simulink model "sampleModel1536"  (R2023a)
settings: Solver=VariableStepAuto  StartTime=0.0  StopTime=10.0  RelTol=1e-3
libraries: hdlsllib x6, simulink x2
settings Model: Creator=user1  LastModifiedBy=user1

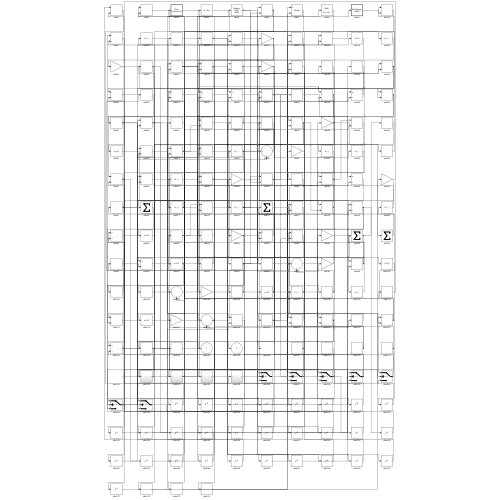
[thumbnail: Simulink's stored preview of the top-level diagram]
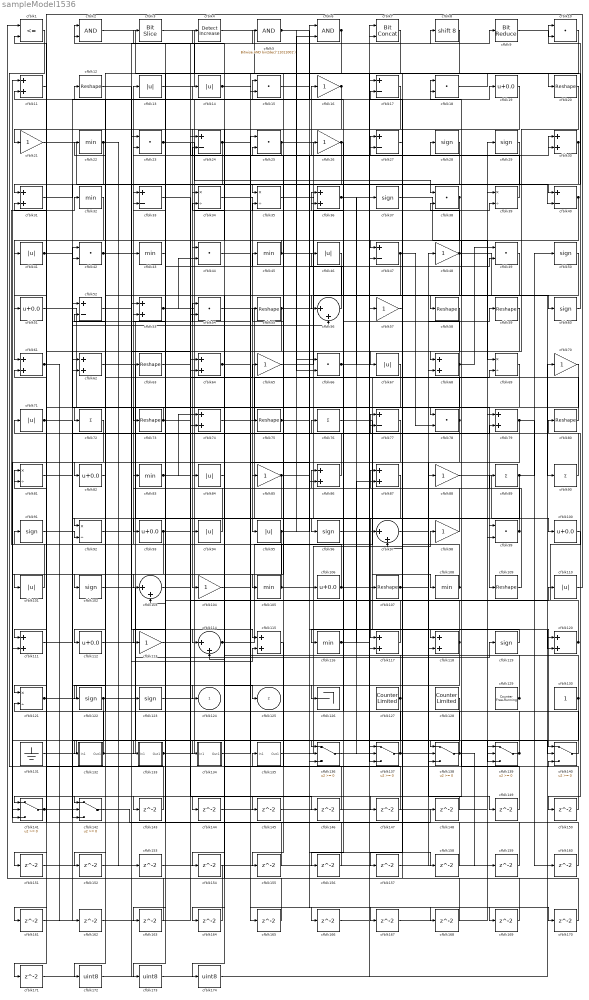
== system sampleModel1536 ==
  cfblk1 : RelationalOperator  Operator=<=  OutDataTypeStr=boolean  InputSameDT=off
  cfblk{10,15,18,23,25,38,42,44,49,54,66,78,99} (13 alike) : DotProduct  OutDataTypeStr=Inherit: Inherit via internal rule
  cfblk{19,51,82,93,100,106,112} (7 alike) : Bias  Bias=0.0  SaturateOnIntegerOverflow=off
  cfblk{13..14,41,46,67,71,84,94..95,101,110} (11 alike) : Abs  SaturateOnIntegerOverflow=off
  cfblk{28..29,37,50,60,91,96,102,119,122..123} (11 alike) : Signum
  cfblk{56,97,103,114} (4 alike) : Sum  Inputs=|++
  cfblk{16,21,26,48,57,65,70,85,88,98,104,113} (12 alike) : Gain
  cfblk{22,32,43,45,83,105,108,116} (8 alike) : MinMax
  cfblk{12,20,55,58..59,63,73,75,80,107,109} (11 alike) : Reshape
  cfblk{11,30..31,36,53,61..62,64,68,74,79,86..87,111,115,117..118,120} (18 alike) : Sum
  cfblk{34..35,39,69,81,92,121} (7 alike) : Product  Inputs=*/  RndMeth=Zero  SaturateOnIntegerOverflow=on
  cfblk126 : Terminator
  cfblk127 : hdlsllib/Sources/Counter Limited  uplimit=7  tsamp=-1
  cfblk128 : hdlsllib/Sources/Counter Limited  uplimit=7  tsamp=-1
  cfblk129 : hdlsllib/Sources/Counter Free-Running  NumBits=16  tsamp=-1
  cfblk130 : Constant  SampleTime=-1
  cfblk131 : Ground
  cfblk132 : Subsystem
      settings: LibrarySourceBlock=|
      | hdlsllib/Ports &
      | Subsystems/Subsystem
  cfblk133 : Subsystem
      settings: LibrarySourceBlock=|
      | hdlsllib/Ports &
      | Subsystems/Subsystem
  cfblk134 : Subsystem
      settings: LibrarySourceBlock=|
      | hdlsllib/Ports &
      | Subsystems/Subsystem
  cfblk135 : Subsystem
      settings: LibrarySourceBlock=|
      | hdlsllib/Ports &
      | Subsystems/Subsystem
  cfblk{136..142} (7 alike) : Switch  SaturateOnIntegerOverflow=off  InputSameDT=off
  cfblk{143..171} (29 alike) : Delay  SampleTime=1
  cfblk{17,24,27,33,40,47,52,77} (8 alike) : Sum  Inputs=+-
  cfblk172 : DataTypeConversion  OutDataTypeStr=uint8  SaturateOnIntegerOverflow=off  RndMeth=Floor
  cfblk173 : DataTypeConversion  OutDataTypeStr=uint8  SaturateOnIntegerOverflow=off  RndMeth=Floor
  cfblk174 : DataTypeConversion  OutDataTypeStr=uint8  SaturateOnIntegerOverflow=off  RndMeth=Floor
  cfblk2 : Logic  AllPortsSameDT=off  OutDataTypeStr=boolean
  cfblk3 : hdlsllib/Logic and Bit Operations/Bit Slice  lidx=7  ridx=0
  cfblk4 : simulink/Logic and Bit Operations/Detect Increase  vinit=0.0  OutDataTypeStr=boolean
      settings: LibrarySourceBlock=|
      | hdlsllib/Logic and Bit
      | Operations/Detect
      | Increase
  cfblk5 : simulink/Logic and Bit Operations/Bitwise Operator  logicop=AND  UseBitMask=on  BitMask=bin2dec('11011001')  BitMaskRealWorld=Stored Integer
      settings: LibrarySourceBlock=|
      | hdlsllib/Logic and Bit
      | Operations/Bitwise
      | Operator
  cfblk6 : Logic  AllPortsSameDT=off  OutDataTypeStr=boolean
  cfblk7 : hdlsllib/Logic and Bit Operations/Bit Concat  numInputs=2
  cfblk{72,76,89..90} (4 alike) : Sum  Inputs=+
  cfblk8 : ArithShift  BitShiftNumber=8
  cfblk9 : hdlsllib/Logic and Bit Operations/Bit Reduce  mode=AND
  cfblk124 : Outport  VectorParamsAs1DForOutWhenUnconnected=off
  cfblk125 : Outport  Port=2  VectorParamsAs1DForOutWhenUnconnected=off
  wires:
  cfblk86/1 -> cfblk71/1
  cfblk34/1 -> cfblk95/1
  cfblk122/1 -> cfblk138/1, cfblk115/2, cfblk171/1
  cfblk101/1 -> cfblk32/1
  cfblk21/1 -> cfblk35/1
  cfblk66/1 -> cfblk37/1, cfblk69/2
  cfblk73/1 -> cfblk72/1, cfblk138/2
  cfblk32/1 -> cfblk111/1
  cfblk39/1 -> cfblk16/1
  cfblk76/1 -> cfblk118/1
  cfblk105/1 -> cfblk13/1, cfblk120/2
  cfblk55/1 -> cfblk78/1, cfblk151/1, cfblk158/1
  cfblk54/1 -> cfblk117/1
  cfblk112/1 -> cfblk119/1
  cfblk20/1 -> cfblk68/1
  cfblk1/1 -> cfblk135/1(In1)
  cfblk2/1 -> cfblk40/1
  cfblk49/1 -> cfblk92/1
  cfblk23/1 -> cfblk38/1, cfblk6/1, cfblk30/2
  cfblk51/1 -> cfblk109/1
  cfblk130/1 -> cfblk142/1, cfblk2/2
  cfblk82/1 -> cfblk12/1
  cfblk96/1 -> cfblk108/1
  cfblk127/1 -> cfblk142/2, cfblk86/1
  cfblk106/1 -> cfblk140/1, cfblk61/2, cfblk46/1
  cfblk78/1 -> cfblk22/1, cfblk152/1
  cfblk135/1(Out1) -> cfblk98/1
  cfblk132/1(Out1) -> cfblk25/1, cfblk81/1
  cfblk47/1 -> cfblk112/1, cfblk78/2, cfblk102/1
  cfblk24/1 -> cfblk82/1, cfblk169/1
  cfblk15/1 -> cfblk106/1
  cfblk133/1(Out1) -> cfblk27/1, cfblk110/1
  cfblk31/1 -> cfblk19/1
  cfblk19/1 -> cfblk93/1
  cfblk25/1 -> cfblk60/1, cfblk24/2
  cfblk87/1 -> cfblk142/3
  cfblk8/1 -> cfblk67/1
  cfblk53/1 -> cfblk35/2, cfblk44/2
  cfblk36/1 -> cfblk107/1, cfblk137/2
  cfblk123/1 -> cfblk15/1
  cfblk45/1 -> cfblk99/1, cfblk41/1
  cfblk67/1 -> cfblk121/1
  cfblk71/1 -> cfblk125/1, cfblk73/1
  cfblk121/1 -> cfblk124/1, cfblk139/3
  cfblk3/1 -> cfblk15/2
  cfblk110/1 -> cfblk21/1
  cfblk62/1 -> cfblk118/2
  cfblk98/1 -> cfblk83/1
  cfblk92/1 -> cfblk4/1
  cfblk69/1 -> cfblk136/1
  cfblk12/1 -> cfblk114/1
  cfblk114/1 -> cfblk48/1, cfblk174/1
  cfblk117/1 -> cfblk91/1
  cfblk29/1 -> cfblk126/1
  cfblk22/1 -> cfblk62/2, cfblk153/1
  cfblk72/1 -> cfblk111/2
  cfblk38/1 -> cfblk61/1, cfblk163/1
  cfblk128/1 -> cfblk141/2
  cfblk5/1 -> cfblk66/2, cfblk170/1
  cfblk11/1 -> cfblk51/1
  cfblk77/1 -> cfblk104/1
  cfblk88/1 -> cfblk100/1
  cfblk59/1 -> cfblk133/1(In1)
  cfblk4/1 -> cfblk137/1
  cfblk113/1 -> cfblk65/1
  cfblk50/1 -> cfblk105/1
  cfblk80/1 -> cfblk63/1
  cfblk75/1 -> cfblk66/1, cfblk77/2, cfblk168/1
  cfblk60/1 -> cfblk10/1
  cfblk18/1 -> cfblk20/1
  cfblk120/1 -> cfblk80/1, cfblk33/1
  cfblk70/1 -> cfblk122/1
  cfblk102/1 -> cfblk136/2
  cfblk27/1 -> cfblk47/1
  cfblk90/1 -> cfblk45/1
  cfblk141/1 -> cfblk42/1, cfblk140/3
  cfblk61/1 -> cfblk161/1, cfblk162/1
  cfblk137/1 -> cfblk88/1, cfblk55/1
  cfblk79/1 -> cfblk138/3, cfblk147/1, cfblk160/1
  cfblk118/1 -> cfblk2/1, cfblk154/1, cfblk155/1
  cfblk97/1 -> cfblk59/1
  cfblk48/1 -> cfblk90/1, cfblk38/2, cfblk144/1
  cfblk74/1 -> cfblk57/1
  cfblk119/1 -> cfblk116/1
  cfblk17/1 -> cfblk31/1
  cfblk6/1 -> cfblk103/1, cfblk85/1
  cfblk134/1(Out1) -> cfblk36/1
  cfblk41/1 -> cfblk75/1, cfblk56/2
  cfblk107/1 -> cfblk87/1, cfblk149/1
  cfblk56/1 -> cfblk3/1
  cfblk26/1 -> cfblk84/1, cfblk56/1
  cfblk35/1 -> cfblk39/2
  cfblk83/1 -> cfblk8/1, cfblk74/1
  cfblk94/1 -> cfblk53/2
  cfblk37/1 -> cfblk69/1
  cfblk16/1 -> cfblk34/1, cfblk44/1
  cfblk13/1 -> cfblk9/1
  cfblk30/1 -> cfblk103/2, cfblk137/3
  cfblk81/1 -> cfblk54/1
  cfblk99/1 -> cfblk94/1, cfblk26/1
  cfblk85/1 -> cfblk77/1, cfblk164/1
  cfblk108/1 -> cfblk28/1, cfblk23/2
  cfblk129/1 -> cfblk76/1, cfblk17/2
  cfblk139/1 -> cfblk97/2, cfblk81/2
  cfblk131/1 -> cfblk140/2
  cfblk93/1 -> cfblk132/1(In1), cfblk5/1
  cfblk64/1 -> cfblk136/3, cfblk86/2
  cfblk9/1 -> cfblk10/2
  cfblk95/1 -> cfblk141/3, cfblk49/2, cfblk6/2, cfblk30/1
  cfblk84/1 -> cfblk14/1
  cfblk52/1 -> cfblk64/2
  cfblk111/1 -> cfblk79/2
  cfblk89/1 -> cfblk113/1, cfblk50/1
  cfblk33/1 -> cfblk96/1
  cfblk103/1 -> cfblk54/2
  cfblk46/1 -> cfblk134/1(In1)
  cfblk140/1 -> cfblk52/2
  cfblk136/1 -> cfblk18/1
  cfblk40/1 -> cfblk58/1, cfblk74/2
  cfblk42/1 -> cfblk115/1, cfblk123/1
  cfblk138/1 -> cfblk36/2, cfblk159/1
  cfblk91/1 -> cfblk92/2
  cfblk28/1 -> cfblk101/1
  cfblk109/1 -> cfblk89/1
  cfblk68/1 -> cfblk11/2, cfblk49/1, cfblk117/2
  cfblk116/1 -> cfblk17/1, cfblk87/2
  cfblk14/1 -> cfblk40/2, cfblk167/1
  cfblk65/1 -> cfblk29/1
  cfblk43/1 -> cfblk143/1
  cfblk143/1 -> cfblk31/2
  cfblk144/1 -> cfblk97/1
  cfblk115/1 -> cfblk145/1
  cfblk145/1 -> cfblk139/1
  cfblk63/1 -> cfblk146/1
  cfblk146/1 -> cfblk34/2
  cfblk147/1 -> cfblk25/2
  cfblk142/1 -> cfblk148/1
  cfblk148/1 -> cfblk141/1
  cfblk149/1 -> cfblk18/2
  cfblk100/1 -> cfblk150/1
  cfblk150/1 -> cfblk120/1
  cfblk151/1 -> cfblk53/1
  cfblk152/1 -> cfblk39/1
  cfblk153/1 -> cfblk79/1
  cfblk154/1 -> cfblk1/1
  cfblk155/1 -> cfblk62/1
  cfblk58/1 -> cfblk156/1
  cfblk156/1 -> cfblk11/1
  cfblk57/1 -> cfblk157/1
  cfblk157/1 -> cfblk68/2
  cfblk158/1 -> cfblk1/2
  cfblk159/1 -> cfblk121/2
  cfblk160/1 -> cfblk33/2
  cfblk161/1 -> cfblk42/2
  cfblk162/1 -> cfblk24/1
  cfblk163/1 -> cfblk23/1
  cfblk164/1 -> cfblk64/1
  cfblk104/1 -> cfblk165/1
  cfblk165/1 -> cfblk52/1
  cfblk44/1 -> cfblk166/1
  cfblk166/1 -> cfblk47/2
  cfblk167/1 -> cfblk99/2
  cfblk168/1 -> cfblk114/2
  cfblk169/1 -> cfblk27/2
  cfblk170/1 -> cfblk139/2
  cfblk171/1 -> cfblk70/1
  cfblk7/1 -> cfblk172/1
  cfblk172/1 -> cfblk43/1
  cfblk10/1 -> cfblk173/1
  cfblk173/1 -> cfblk7/1
  cfblk174/1 -> cfblk7/2

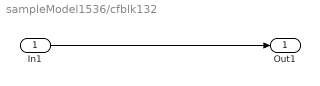
== system sampleModel1536/cfblk132 ==
  In1 : Inport
  Out1 : Outport
  wires:
  In1/1 -> Out1/1

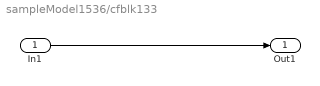
== system sampleModel1536/cfblk133 ==
  In1 : Inport
  Out1 : Outport
  wires:
  In1/1 -> Out1/1

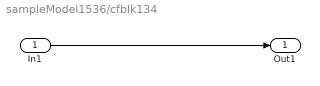
== system sampleModel1536/cfblk134 ==
  In1 : Inport
  Out1 : Outport
  wires:
  In1/1 -> Out1/1

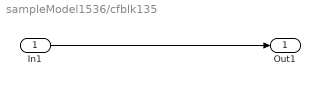
== system sampleModel1536/cfblk135 ==
  In1 : Inport
  Out1 : Outport
  wires:
  In1/1 -> Out1/1
